simulink model "roundabout_onthego_path"  (R2016b)
settings: Solver=FixedStepAuto  StartTime=0.0  StopTime=inf  RelTol=1e-3
undefined symbols (not defined in the file): DiscIntNeverNeededParam, vehicle_name
libraries: simulink x8, SCANeR_API x6
(part 1 of 2)
settings Model: Creator=z041288  LastModifiedBy=z041288

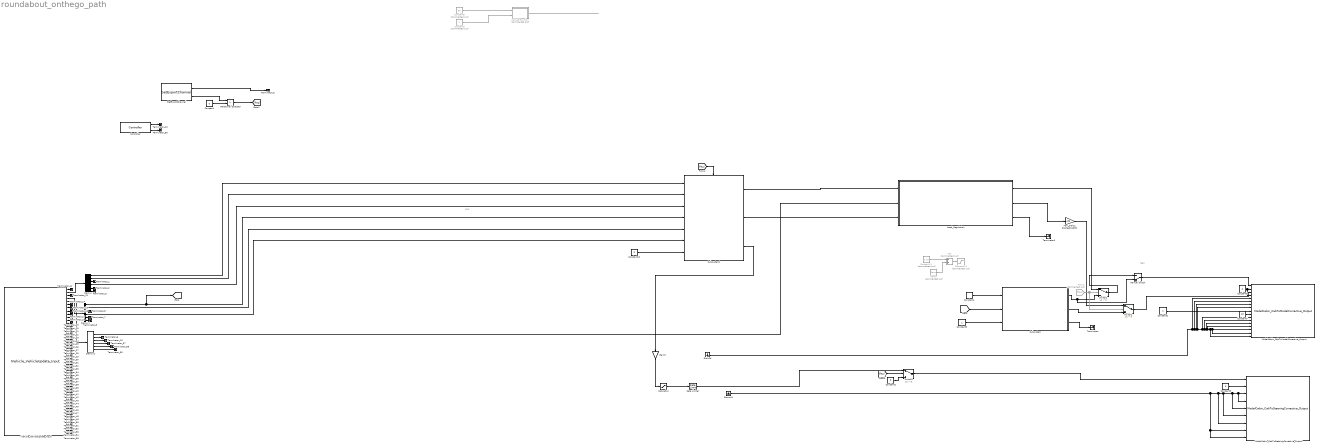
== system roundabout_onthego_path ==
  note: yaw
  note: Man
  Accel_Regulation : Subsystem
  Add : Sum  Commented=on
  Constant{,1,3,6} (4 alike) : Constant  Value=0
  Constant10 : Constant  Value=2
  Constant11 : Constant  Commented=on  Value=2.78
  Constant2 : Constant
  Constant4 : Constant  Value=10*5/18
  Constant5 : Constant
  Constant7 : Constant  Value=10
  Constant8 : Constant  Commented=on  Value=50
  Constant9 : Constant  Commented=on  Value=4
  Controller : SCANeR_API/Controller  Priority=1  Config='NEWCONFIG_Training'  ProcName='SIMULINK'  Frequency=100  NetworkOutputFrequency=100  TimeOut=3000  IsSynchronized=on
  Demux : Demux  Outputs=6
  Demux1 : Demux  Outputs=6
  Demux2 : Demux  Outputs=6
  From2 : From  Commented=on  GotoTag=flag
  Gain3 : Gain  Gain=1/57
  GetExportChannel : SCANeR_API/GetExportChannel  Priority=0  ExportChannelCategory='debug'  ExportChannelName='SF_debug_001'  VehicleId=-1
  Ground : Ground
  Ground1 : Ground
  IVehicle_VehicleUpdate_Input : SCANeR_API/Network inputs/IVehicle/IVehicle_VehicleUpdate_Input  Priority=2  ev=off  vhlId=0
  MATLAB Function : MATLAB Function  Commented=on  TreatAsAtomicUnit=on
  Manual Switch : ManualSwitch  CurrentSetting=0
  Max_brake_SCANeR=400N : Gain  Gain=400
  ModelCabin_CabToModelCorrective_Output : SCANeR_API/SHM outputs/ModelCabin/ModelCabin_CabToModelCorrective_Output  Priority=2  shmId=0
  ModelCabin_CabToSteeringCorrective_Output : SCANeR_API/SHM outputs/ModelCabin/ModelCabin_CabToSteeringCorrective_Output  Priority=2  shmId=0
  Ramp : simulink/Sources/Ramp  Commented=on  slope=25/30  start=0  X0=0
  Rate Limiter : RateLimiter  RisingSlewLimit=10  FallingSlewLimit=-10  SampleTimeMode=inherited
  Relational Operator : RelationalOperator  Operator=>  OutDataTypeStr=boolean  RndMeth=Simplest
  Saturation : Saturate  UpperLimit=10  LowerLimit=-10
  Saturation1 : Saturate  Commented=on  UpperLimit=75/18  LowerLimit=0
  Subsystem : Subsystem
  Subsystem1 : Subsystem
  Switch1 : Switch  Criteria=u2 > Threshold  Threshold=5
  Switch2 : Switch  Criteria=u2 > Threshold
  Switch3 : Switch  Criteria=u2 > Threshold
  Terminator : Terminator
  Terminator1 : Terminator
  Terminator_{1..3,5..59} (58 alike) : Terminator
  wires:
  GetExportChannel/1 -> Terminator_9/1
  GetExportChannel/2 -> Relational Operator/1
  Constant/1 -> Relational Operator/2
  Controller/1 -> Terminator_10/1
  Controller/2 -> Terminator_56/1
  IVehicle_VehicleUpdate_Input/2 -> Demux/1
  IVehicle_VehicleUpdate_Input/4 -> Demux1/1
  Gain3/1 -> Saturation/1
  Ground1/1 -> ModelCabin_CabToSteeringCorrective_Output/8, ModelCabin_CabToSteeringCorrective_Output/9, ModelCabin_CabToSteeringCorrective_Output/4, ModelCabin_CabToSteeringCorrective_Output/3, ModelCabin_CabToSteeringCorrective_Output/5, ModelCabin_CabToSteeringCorrective_Output/6, ModelCabin_CabToSteeringCorrective_Output/7
  Demux/3 -> Terminator_1/1
  Demux/5 -> Terminator_2/1
  Demux/6 -> Terminator_3/1
  Demux1/3 -> Terminator_5/1
  Demux1/5 -> Terminator_7/1
  Demux1/6 -> Terminator_8/1
  IVehicle_VehicleUpdate_Input/1 -> Terminator_11/1
  IVehicle_VehicleUpdate_Input/3 -> Terminator_12/1
  IVehicle_VehicleUpdate_Input/5 -> Demux2/1
  IVehicle_VehicleUpdate_Input/6 -> Terminator_14/1
  IVehicle_VehicleUpdate_Input/7 -> Terminator_15/1
  IVehicle_VehicleUpdate_Input/8 -> Terminator_16/1
  IVehicle_VehicleUpdate_Input/9 -> Terminator_17/1
  IVehicle_VehicleUpdate_Input/10 -> Terminator_18/1
  IVehicle_VehicleUpdate_Input/11 -> Terminator_19/1
  IVehicle_VehicleUpdate_Input/12 -> Terminator_20/1
  IVehicle_VehicleUpdate_Input/13 -> Terminator_21/1
  IVehicle_VehicleUpdate_Input/14 -> Terminator_22/1
  IVehicle_VehicleUpdate_Input/15 -> Terminator_23/1
  IVehicle_VehicleUpdate_Input/16 -> Terminator_24/1
  IVehicle_VehicleUpdate_Input/17 -> Terminator_25/1
  IVehicle_VehicleUpdate_Input/18 -> Terminator_26/1
  IVehicle_VehicleUpdate_Input/19 -> Terminator_27/1
  IVehicle_VehicleUpdate_Input/20 -> Terminator_28/1
  IVehicle_VehicleUpdate_Input/21 -> Terminator_29/1
  IVehicle_VehicleUpdate_Input/22 -> Terminator_30/1
  IVehicle_VehicleUpdate_Input/23 -> Terminator_31/1
  IVehicle_VehicleUpdate_Input/24 -> Terminator_32/1
  IVehicle_VehicleUpdate_Input/25 -> Terminator_33/1
  IVehicle_VehicleUpdate_Input/26 -> Terminator_34/1
  IVehicle_VehicleUpdate_Input/27 -> Terminator_35/1
  IVehicle_VehicleUpdate_Input/28 -> Terminator_36/1
  IVehicle_VehicleUpdate_Input/29 -> Terminator_37/1
  IVehicle_VehicleUpdate_Input/30 -> Terminator_38/1
  IVehicle_VehicleUpdate_Input/31 -> Terminator_39/1
  IVehicle_VehicleUpdate_Input/32 -> Terminator_40/1
  IVehicle_VehicleUpdate_Input/33 -> Terminator_41/1
  IVehicle_VehicleUpdate_Input/34 -> Terminator_42/1
  IVehicle_VehicleUpdate_Input/35 -> Terminator_43/1
  IVehicle_VehicleUpdate_Input/36 -> Terminator_44/1
  IVehicle_VehicleUpdate_Input/37 -> Terminator_45/1
  IVehicle_VehicleUpdate_Input/38 -> Terminator_46/1
  IVehicle_VehicleUpdate_Input/39 -> Terminator_47/1
  IVehicle_VehicleUpdate_Input/40 -> Terminator_48/1
  IVehicle_VehicleUpdate_Input/41 -> Terminator_49/1
  IVehicle_VehicleUpdate_Input/42 -> Terminator_50/1
  IVehicle_VehicleUpdate_Input/43 -> Terminator_51/1
  IVehicle_VehicleUpdate_Input/44 -> Terminator_52/1
  IVehicle_VehicleUpdate_Input/45 -> Terminator_53/1
  IVehicle_VehicleUpdate_Input/46 -> Terminator_54/1
  IVehicle_VehicleUpdate_Input/47 -> Terminator_55/1
  Ground/1 -> ModelCabin_CabToModelCorrective_Output/5, ModelCabin_CabToModelCorrective_Output/6, ModelCabin_CabToModelCorrective_Output/7, ModelCabin_CabToModelCorrective_Output/8, ModelCabin_CabToModelCorrective_Output/11, ModelCabin_CabToModelCorrective_Output/12, ModelCabin_CabToModelCorrective_Output/13, ModelCabin_CabToModelCorrective_Output/14, ModelCabin_CabToModelCorrective_Output/17, ModelCabin_CabToModelCorrective_Output/16, ModelCabin_CabToModelCorrective_Output/15
  Demux1/1 -> Subsystem1/4(xd_in), [speed]  "vlongi"
  Saturation/1 -> Rate Limiter/1
  Demux2/1 -> Accel_Regulation/2(Vehicle_accel_[m/s2])
  Accel_Regulation/2(brake [0_1]) -> Max_brake_SCANeR=400N/1
  Demux2/2 -> Terminator_6/1
  Demux2/3 -> Terminator_13/1
  Demux2/4 -> Terminator_57/1
  Demux2/5 -> Terminator_58/1
  Demux2/6 -> Terminator_59/1
  Constant2/1 -> ModelCabin_CabToModelCorrective_Output/9
  Constant3/1 -> ModelCabin_CabToSteeringCorrective_Output/2
  Constant5/1 -> Subsystem/3(Speed_control_on)
  [speed] -> Subsystem/2(Vehicle_Speed_[m/s])
  Accel_Regulation/1(accel [0_1]) -> Switch1/1
  Subsystem/1(accel_regul [0_1]) -> Manual Switch/2, Switch1/3
  Switch1/1 -> Manual Switch/1
  Constant6/1 -> ModelCabin_CabToModelCorrective_Output/4, ModelCabin_CabToModelCorrective_Output/2
  Constant7/1 -> ModelCabin_CabToModelCorrective_Output/10
  Max_brake_SCANeR=400N/1 -> Switch2/1
  Subsystem/2(Driver_Brake [0_1]) -> Switch2/3
  Switch2/1 -> ModelCabin_CabToModelCorrective_Output/3
  Relational Operator/1 -> [flag]
  From2/1 -> Switch1/2, Switch2/2
  Subsystem/3(Gear_d) -> Terminator/1
  Accel_Regulation/3(Gear_d) -> Terminator1/1
  Demux/1 -> Subsystem1/1(x_in)  "x"
  Demux/2 -> Subsystem1/2(y_in)  "y"
  Demux/4 -> Subsystem1/3(yaw_in)  "yaw"
  Demux1/2 -> Subsystem1/5(yd_in)  "vlat"
  Demux1/4 -> Subsystem1/6(yawd_in)  "yawdot"
  Subsystem1/1(Out11) -> Accel_Regulation/1(Intended_Vehicle_accel_[m/s2])
  Subsystem1/2(Out12) -> Accel_Regulation/3(Accel_control_on)
  Subsystem1/3(Out13) -> Gain3/1
  [flag] -> Subsystem1/Enable
  Rate Limiter/1 -> Switch3/1
  Switch3/1 -> ModelCabin_CabToSteeringCorrective_Output/1
  [flag] -> Switch3/2
  Constant1/1 -> Switch3/3
  Constant9/1 -> MATLAB Function/2(exit)
  Constant8/1 -> MATLAB Function/1(r)
  MATLAB Function/1(y) -> ?
  Constant10/1 -> Subsystem1/7(Maneuver)
  Manual Switch/1 -> ModelCabin_CabToModelCorrective_Output/1
  Ramp/1 -> Add/2
  Add/1 -> Saturation1/1
  Constant11/1 -> Add/1
  Constant4/1 -> Subsystem/1(Intended_Vehicle_Speed_[m/s])

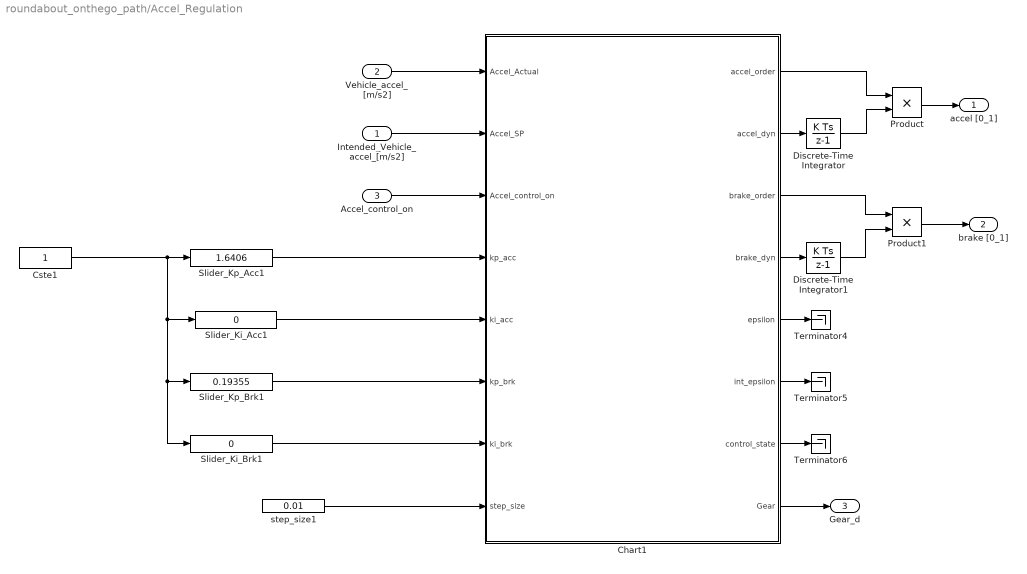
== system roundabout_onthego_path/Accel_Regulation ==
  Intended_Vehicle_accel_[m/s2] : Inport
  Vehicle_accel_[m/s2] : Inport  Port=2
  Accel_control_on : Inport  Port=3
  Chart1 : Stateflow chart  TreatAsAtomicUnit=on  SystemSampleTime=0.01
  Cste1 : Constant  SampleTime=0.01
  Discrete-Time Integrator : DiscreteIntegrator  SampleTime=-1  LimitOutput=on  UpperSaturationLimit=1  LowerSaturationLimit=0  ICPrevOutput=DiscIntNeverNeededParam  ICPrevScaledInput=DiscIntNeverNeededParam
  Discrete-Time Integrator1 : DiscreteIntegrator  SampleTime=-1  LimitOutput=on  UpperSaturationLimit=1  LowerSaturationLimit=0  ICPrevOutput=DiscIntNeverNeededParam  ICPrevScaledInput=DiscIntNeverNeededParam
  Product : Product
  Product1 : Product
  Slider_Ki_Acc1 : simulink/Math Operations/Slider Gain  low=0  gain=0  high=2
  Slider_Ki_Brk1 : simulink/Math Operations/Slider Gain  low=0  gain=0  high=2
  Slider_Kp_Acc1 : simulink/Math Operations/Slider Gain  low=0  gain=1.6406  high=10
  Slider_Kp_Brk1 : simulink/Math Operations/Slider Gain  low=0  gain=0.19355  high=2
  Terminator4 : Terminator
  Terminator5 : Terminator
  Terminator6 : Terminator
  step_size1 : Constant  Value=0.01  SampleTime=0.01
  accel [0_1] : Outport
  brake [0_1] : Outport  Port=2
  Gear_d : Outport  Port=3
  wires:
  Intended_Vehicle_accel_[m/s2]/1 -> Chart1/2(Accel_SP)
  Vehicle_accel_[m/s2]/1 -> Chart1/1(Accel_Actual)
  Accel_control_on/1 -> Chart1/3(Accel_control_on)
  step_size1/1 -> Chart1/8(step_size)
  Chart1/5(epsilon) -> Terminator4/1
  Chart1/6(int_epsilon) -> Terminator5/1
  Slider_Kp_Acc1/1 -> Chart1/4(kp_acc)
  Slider_Ki_Acc1/1 -> Chart1/5(ki_acc)
  Slider_Ki_Brk1/1 -> Chart1/7(ki_brk)
  Slider_Kp_Brk1/1 -> Chart1/6(kp_brk)
  Cste1/1 -> Slider_Ki_Acc1/1, Slider_Kp_Brk1/1, Slider_Ki_Brk1/1, Slider_Kp_Acc1/1
  Chart1/4(brake_dyn) -> Discrete-Time Integrator1/1
  Chart1/2(accel_dyn) -> Discrete-Time Integrator/1
  Chart1/1(accel_order) -> Product/1
  Discrete-Time Integrator/1 -> Product/2
  Product/1 -> accel [0_1]/1
  Chart1/3(brake_order) -> Product1/1
  Discrete-Time Integrator1/1 -> Product1/2
  Product1/1 -> brake [0_1]/1
  Chart1/7(control_state) -> Terminator6/1
  Chart1/8(Gear) -> Gear_d/1

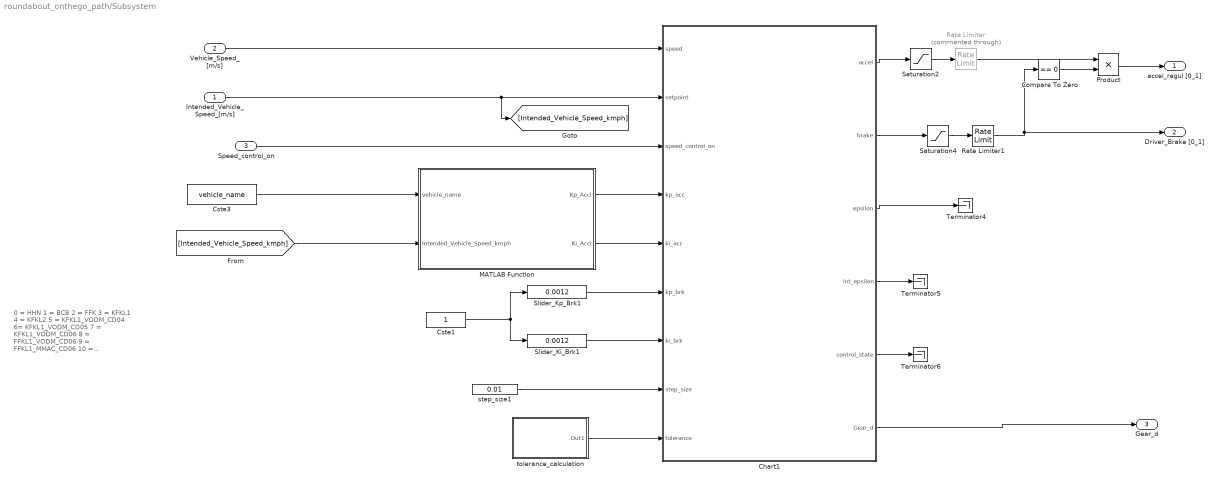
== system roundabout_onthego_path/Subsystem ==
  note: 0 = HHN
      | 1 = BCB
      | 2 = FFK
      | 3 = KFKL1
      | 4 = KFKL2
      | 5 = KFKL1_VODM_CD04
      | 6= KFKL1_VODM_CD05
      | 7 = KFKL1_VODM_CD06
      | 8 = FFKL1_VODM_CD06
      | 9 = FFKL1_MMAC_CD06
      | 10 = FFKL2_MMAC_CD06
      | 11 = KFKL2_MMAC_CD06
      | 12 = XDD_35T_TRS_L2H2
  Intended_Vehicle_Speed_[m/s] : Inport
  Vehicle_Speed_[m/s] : Inport  Port=2
  Speed_control_on : Inport  Port=3
  Chart1 : Stateflow chart  TreatAsAtomicUnit=on  SystemSampleTime=0.01
  Compare To Zero : simulink/Logic and Bit Operations/Compare To Zero  relop===  OutDataTypeStr=boolean
  Cste1 : Constant  SampleTime=0.01
  Cste3 : Constant  Value=vehicle_name  SampleTime=0.01
  MATLAB Function : MATLAB Function  TreatAsAtomicUnit=on
  Product : Product
  Rate Limiter : RateLimiter  Commented=through  RisingSlewLimit=0.5  SampleTimeMode=inherited
  Rate Limiter1 : RateLimiter  RisingSlewLimit=0.2  SampleTimeMode=inherited
  Saturation2 : Saturate  UpperLimit=1  LowerLimit=0  SampleTime=0.01
  Saturation4 : Saturate  UpperLimit=1  LowerLimit=0  SampleTime=0.01
  Slider_Ki_Brk1 : simulink/Math Operations/Slider Gain  low=0  gain=0.0012  high=2
  Slider_Kp_Brk1 : simulink/Math Operations/Slider Gain  low=0  gain=0.0012  high=1
  Terminator4 : Terminator
  Terminator5 : Terminator
  Terminator6 : Terminator
  step_size1 : Constant  Value=0.01  SampleTime=0.01
  tolerance_calculation : Subsystem
  accel_regul [0_1] : Outport
  Driver_Brake [0_1] : Outport  Port=2
  Gear_d : Outport  Port=3
  wires:
  Cste1/1 -> Slider_Kp_Brk1/1, Slider_Ki_Brk1/1
  Slider_Kp_Brk1/1 -> Chart1/6(kp_brk)
  Slider_Ki_Brk1/1 -> Chart1/7(ki_brk)
  MATLAB Function/2(Ki_Accl) -> Chart1/5(ki_acc)
  MATLAB Function/1(Kp_Accl) -> Chart1/4(kp_acc)
  Chart1/5(control_state) -> Terminator6/1
  Chart1/4(int_epsilon) -> Terminator5/1
  Chart1/3(epsilon) -> Terminator4/1
  Chart1/2(brake) -> Saturation4/1
  step_size1/1 -> Chart1/8(step_size)
  Saturation4/1 -> Rate Limiter1/1
  Vehicle_Speed_[m/s]/1 -> Chart1/1(speed)
  Intended_Vehicle_Speed_[m/s]/1 -> [Intended_Vehicle_Speed_kmph], Chart1/2(setpoint)
  Saturation2/1 -> Rate Limiter/1
  Rate Limiter/1 -> Product/1
  Product/1 -> accel_regul [0_1]/1
  Rate Limiter1/1 -> Compare To Zero/1, Driver_Brake [0_1]/1
  Chart1/6(Gear_d) -> Gear_d/1
  Speed_control_on/1 -> Chart1/3(speed_control_on)
  Cste3/1 -> MATLAB Function/1(vehicle_name)
  [Intended_Vehicle_Speed_kmph] -> MATLAB Function/2(Intended_Vehicle_Speed_kmph)
  Compare To Zero/1 -> Product/2
  Chart1/1(accel) -> Saturation2/1
  tolerance_calculation/1(Out1) -> Chart1/9(tolerance)

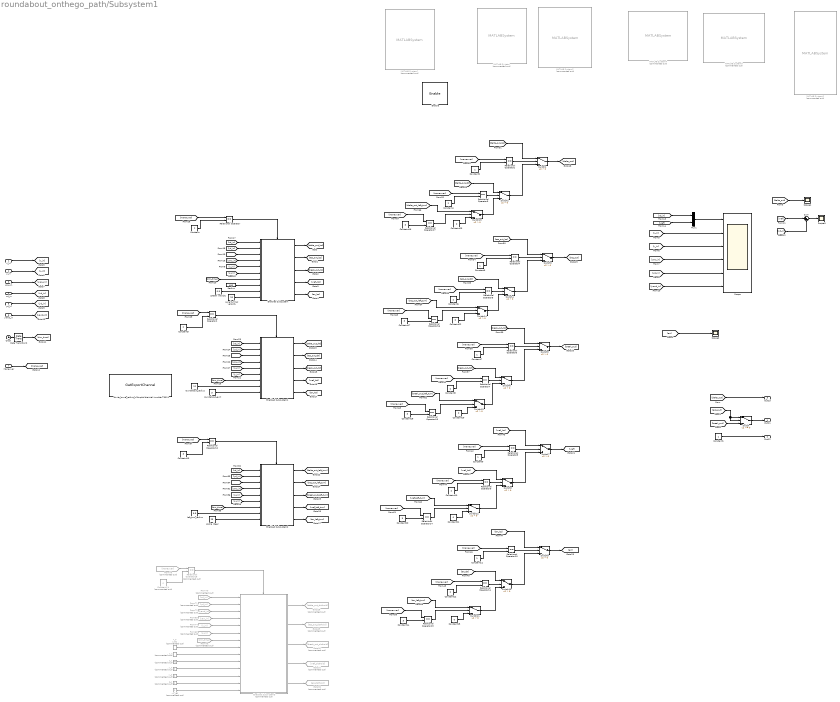
== system roundabout_onthego_path/Subsystem1 ==
  x_in : Inport
  y_in : Inport  Port=2
  yaw_in : Inport  Port=3
  xd_in : Inport  Port=4
  yd_in : Inport  Port=5
  yawd_in : Inport  Port=6
  Maneuver : Inport  Port=7
  Enable : EnablePort  PropagateVarSize=During execution
  Clock : Clock
  Constant{,1..2,5,7,9,11} (7 alike) : Constant
  Constant{3..4,6,8,10,12} (6 alike) : Constant  Value=2
  Constant{13..14,16..18,20} (6 alike) : Constant  Value=3
  Constant{15,19,21..23} (5 alike) : Constant  Value=0
  Constant24 : Constant  Commented=on  Value=4
  Enabled Subsystem : Subsystem  TreatAsAtomicUnit=on
  Enabled Subsystem1 : Subsystem  TreatAsAtomicUnit=on
  Enabled Subsystem2 : Subsystem  TreatAsAtomicUnit=on
  Enabled Subsystem3 : Subsystem  Commented=on  TreatAsAtomicUnit=on
  From68 : From  Commented=on  GotoTag=y_in
  From69 : From  Commented=on  GotoTag=yaw_in
  From70 : From  Commented=on  GotoTag=xd_in
  From71 : From  Commented=on  GotoTag=yd_in
  From72 : From  Commented=on  GotoTag=yawd_in
  From73 : From  Commented=on  GotoTag=sim_time
  From74 : From  Commented=on  GotoTag=x_in
  From75 : From  Commented=on  GotoTag=maneuver
  Goto28 : Goto  Commented=on  GotoTag=delta_out_clothoid
  Goto29 : Goto  Commented=on  GotoTag=acc_out_clothoid
  Goto30 : Goto  Commented=on  GotoTag=break_out_clothoid
  Goto31 : Goto  Commented=on  GotoTag=vref_clothoid
  Goto32 : Goto  Commented=on  GotoTag=err_clothoid
  Lateral velocity : Constant  Value=0.5
  Longitudinal velocity : Constant  Value=20
  MATLAB System : MATLABSystem  Commented=on  System=casadi_block_MPCtry_1  SimulateUsing=Interpreted execution
      mask Type: casadi_block_MPCtry_1
      mask Display:
      | disp('casadi_block_MPCtry_1');
      | port_label('input',1,'xd_in');
      | port_label('input',2,'yd_in');
      | port_label('input',3,'yawd_in');
      | port_label('input',4,'yaw_in');
      | port_label('input',5,'x_in');
      | port_label('input',6,'y_in');
      | port_label('input',7,'t');
      | port_label('output',1,'delta_out');
      | port_label('output',2,'acc_out');
      | port_label('output',3,'break_out');
      | port_label('output',4,'vref');
      | port_label('output',5,'err');
  MATLAB System1 : MATLABSystem  Commented=on  System=casadi_block_MPCtry_3  SimulateUsing=Interpreted execution
      mask Type: casadi_block_MPCtry_3
      mask Display:
      | disp('casadi_block_MPCtry_3');
      | port_label('input',1,'xd_in');
      | port_label('input',2,'yd_in');
      | port_label('input',3,'yawd_in');
      | port_label('input',4,'yaw_in');
      | port_label('input',5,'x_in');
      | port_label('input',6,'y_in');
      | port_label('input',7,'t');
      | port_label('output',1,'delta_out');
      | port_label('output',2,'acc_out');
      | port_label('output',3,'break_out');
      | port_label('output',4,'vref');
      | port_label('output',5,'err');
  MATLAB System2 : MATLABSystem  Commented=on  System=casadi_block_MPC_LSS  SimulateUsing=Interpreted execution
      mask Type: casadi_block_MPC_LSS
      mask Display:
      | disp('casadi_block_MPC_LSS');
      | port_label('input',1,'xd_in');
      | port_label('input',2,'yd_in');
      | port_label('input',3,'yawd_in');
      | port_label('input',4,'yaw_in');
      | port_label('input',5,'x_in');
      | port_label('input',6,'y_in');
      | port_label('input',7,'t');
      | port_label('output',1,'delta_out');
      | port_label('output',2,'acc_out');
      | port_label('output',3,'break_out');
      | port_label('output',4,'vref');
      | port_label('output',5,'err');
  MATLAB System3 : MATLABSystem  Commented=on  System=casadi_block_MPC_left_turn  SimulateUsing=Interpreted execution
      mask Type: casadi_block_MPC_left_turn
      mask Display:
      | disp('casadi_block_MPC_left_turn');
      | port_label('input',1,'xd_in');
      | port_label('input',2,'yd_in');
      | port_label('input',3,'yawd_in');
      | port_label('input',4,'yaw_in');
      | port_label('input',5,'x_in');
      | port_label('input',6,'y_in');
      | port_label('input',7,'t');
      | port_label('output',1,'delta_out');
      | port_label('output',2,'acc_out');
      | port_label('output',3,'break_out');
      | port_label('output',4,'vref');
      | port_label('output',5,'err');
  MATLAB System4 : MATLABSystem  Commented=on  System=casadi_block_MPC_left_turn_2  SimulateUsing=Interpreted execution
      mask Type: casadi_block_MPC_left_turn_2
      mask Display:
      | disp('casadi_block_MPC_left_turn_2');
      | port_label('input',1,'xd_in');
      | port_label('input',2,'yd_in');
      | port_label('input',3,'yawd_in');
      | port_label('input',4,'yaw_in');
      | port_label('input',5,'x_in');
      | port_label('input',6,'y_in');
      | port_label('input',7,'t');
      | port_label('output',1,'delta_out');
      | port_label('output',2,'acc_out');
      | port_label('output',3,'break_out');
      | port_label('output',4,'vref');
      | port_label('output',5,'err');
  MATLAB System5 : MATLABSystem  Commented=on  System=casadi_block_MPCtry_4  SimulateUsing=Interpreted execution
      mask Type: casadi_block_MPCtry_4
      mask Display:
      | disp('casadi_block_MPCtry_4');
      | port_label('input',1,'xd_in');
      | port_label('input',2,'yd_in');
      | port_label('input',3,'yawd_in');
      | port_label('input',4,'yaw_in');
      | port_label('input',5,'x_in');
      | port_label('input',6,'y_in');
      | port_label('input',7,'t');
      | port_label('input',8,'ref_path');
      | port_label('output',1,'delta_out');
      | port_label('output',2,'acc_out');
      | port_label('output',3,'break_out');
      | port_label('output',4,'vref');
      | port_label('output',5,'err');
  Mux1 : Mux  Inputs=2
  Radius : Constant  Value=400
  Rate Transition2 : RateTransition  OutPortSampleTime=0.02
  Relational Operator{,1..17} (18 alike) : RelationalOperator  Operator===  OutDataTypeStr=boolean  RndMeth=Simplest
  Relational Operator18 : RelationalOperator  Commented=on  Operator===  OutDataTypeStr=boolean  RndMeth=Simplest
  Scope : Scope  NumInputPorts=6
  Scope1 : Scope
  Scope2 : Scope
  Scope3 : Scope
  Sum : Sum  Inputs=|+-
  Switch : Switch
  Switch{1..15} (15 alike) : Switch  Criteria=u2 > Threshold
  alpha (deg) : Constant  Value=23
  driver_curve_radius_m export channel number - 6011 : SCANeR_API/GetExportChannel  Priority=0  ExportChannelCategory='system'  ExportChannelName='driver_curve_radius_m'  VehicleId=-1
  left_turn_radius : Constant  Value=9.5
  roundabout_exit : Constant  Value=3
  roundabout_radius : Constant  Value=12
  t_o : Constant  Commented=on
  t_s : Constant  Commented=on  Value=90
  vv_ref : Constant  Commented=on
  x_o : Constant  Commented=on
  x_s : Constant  Commented=on  Value=1.82
  y_o : Constant  Commented=on
  y_s : Constant  Commented=on  Value=-60
  Out11 : Outport
  Out12 : Outport  Port=2
  Out13 : Outport  Port=3
  wires:
  [x_in] -> Scope/2
  [y_in] -> Scope/3
  [yawd_in] -> Scope/6
  [yd_in] -> Scope/5
  [err] -> Scope2/1
  Rate Transition2/1 -> [sim_time]
  Mux1/1 -> Scope/1
  [acc_out] -> Switch/2, Switch/1
  Clock/1 -> Rate Transition2/1
  [yaw_in] -> Scope/4
  Switch/1 -> Out11/1
  [break_out] -> Switch/3
  Sum/1 -> Scope3/1
  Constant1/1 -> Out12/1
  roundabout_radius/1 -> Enabled Subsystem1/8(In8)
  roundabout_exit/1 -> Enabled Subsystem1/9(In9)
  Enabled Subsystem/1(Out1) -> [delta_out_lss]
  Enabled Subsystem/2(Out2) -> [acc_out_lss]
  Enabled Subsystem/3(Out3) -> [break_out_lss]
  Enabled Subsystem/4(Out4) -> [vref_lss]
  Enabled Subsystem/5(Out5) -> [err_lss]
  x_in/1 -> [x_in]
  y_in/1 -> [y_in]
  yaw_in/1 -> [yaw_in]
  xd_in/1 -> [xd_in]
  yd_in/1 -> [yd_in]
  yawd_in/1 -> [yawd_in]
  [vref] -> Sum/1
  [xd_in] -> Sum/2
  [xd_in] -> Mux1/1
  [vref] -> Mux1/2
  [delta_out] -> Out13/1
  [x_in] -> Enabled Subsystem/5(In5)
  [y_in] -> Enabled Subsystem/6(In6)
  [yaw_in] -> Enabled Subsystem/4(In4)
  [xd_in] -> Enabled Subsystem/1(In1)
  [yd_in] -> Enabled Subsystem/2(In2)
  [yawd_in] -> Enabled Subsystem/3(In3)
  [sim_time] -> Enabled Subsystem/7(In7)
  [x_in] -> Enabled Subsystem1/5(In5)
  [y_in] -> Enabled Subsystem1/6(In6)
  [yaw_in] -> Enabled Subsystem1/4(In4)
  [xd_in] -> Enabled Subsystem1/1(In1)
  [yd_in] -> Enabled Subsystem1/2(In2)
  [yawd_in] -> Enabled Subsystem1/3(In3)
  [sim_time] -> Enabled Subsystem1/7(In7)
  Maneuver/1 -> [maneuver]
  [maneuver] -> Relational Operator/1
  Constant/1 -> Relational Operator/2
  Constant3/1 -> Relational Operator1/2
  [maneuver] -> Relational Operator1/1
  Relational Operator/1 -> Enabled Subsystem/Enable
  Relational Operator1/1 -> Enabled Subsystem1/Enable
  Enabled Subsystem1/1(Out1) -> [delta_out_rbt]
  Enabled Subsystem1/2(Out2) -> [acc_out_rbt]
  Enabled Subsystem1/3(Out3) -> [break_out_rbt]
  Enabled Subsystem1/4(Out4) -> [vref_rbt]
  Enabled Subsystem1/5(Out5) -> [err_rbt]
  [maneuver] -> Relational Operator2/1
  Constant2/1 -> Relational Operator2/2
  Relational Operator2/1 -> Switch1/2
  [delta_out_lss] -> Switch1/1
  [maneuver] -> Relational Operator3/1
  Constant4/1 -> Relational Operator3/2
  Relational Operator3/1 -> Switch2/2
  Switch2/1 -> Switch1/3
  [delta_out_rbt] -> Switch2/1
  Switch1/1 -> [delta_out]
  [maneuver] -> Relational Operator4/1
  Constant5/1 -> Relational Operator4/2
  Relational Operator4/1 -> Switch3/2
  [acc_out_lss] -> Switch3/1
  [maneuver] -> Relational Operator5/1
  Constant6/1 -> Relational Operator5/2
  Relational Operator5/1 -> Switch4/2
  Switch4/1 -> Switch3/3
  [acc_out_rbt] -> Switch4/1
  Switch3/1 -> [acc_out]
  [maneuver] -> Relational Operator6/1
  Constant7/1 -> Relational Operator6/2
  Relational Operator6/1 -> Switch5/2
  [break_out_lss] -> Switch5/1
  [maneuver] -> Relational Operator7/1
  Constant8/1 -> Relational Operator7/2
  Relational Operator7/1 -> Switch6/2
  Switch6/1 -> Switch5/3
  [break_out_rbt] -> Switch6/1
  Switch5/1 -> [break_out]
  [maneuver] -> Relational Operator8/1
  Constant9/1 -> Relational Operator8/2
  Relational Operator8/1 -> Switch7/2
  [vref_lss] -> Switch7/1
  [maneuver] -> Relational Operator9/1
  Constant10/1 -> Relational Operator9/2
  Relational Operator9/1 -> Switch8/2
  Switch8/1 -> Switch7/3
  [vref_rbt] -> Switch8/1
  Switch7/1 -> [vref]
  [maneuver] -> Relational Operator10/1
  Constant11/1 -> Relational Operator10/2
  Relational Operator10/1 -> Switch9/2
  [err_lss] -> Switch9/1
  [maneuver] -> Relational Operator11/1
  Constant12/1 -> Relational Operator11/2
  Relational Operator11/1 -> Switch10/2
  Switch10/1 -> Switch9/3
  [err_rbt] -> Switch10/1
  Switch9/1 -> [err]
  Radius/1 -> Enabled Subsystem/8(In8)
  Lateral velocity/1 -> Enabled Subsystem/9(In9)
  Longitudinal velocity/1 -> Enabled Subsystem/10(In10)
  Switch15/1 -> Switch2/3
  Switch14/1 -> Switch4/3
  Switch13/1 -> Switch6/3
  Switch12/1 -> Switch8/3
  Switch11/1 -> Switch10/3
  [delta_out] -> Scope1/1
  left_turn_radius/1 -> Enabled Subsystem2/8(In8)
  alpha (deg)/1 -> Enabled Subsystem2/9(In9)
  [x_in] -> Enabled Subsystem2/5(In5)
  [y_in] -> Enabled Subsystem2/6(In6)
  [yaw_in] -> Enabled Subsystem2/4(In4)
  [xd_in] -> Enabled Subsystem2/1(In1)
  [yd_in] -> Enabled Subsystem2/2(In2)
  [yawd_in] -> Enabled Subsystem2/3(In3)
  [sim_time] -> Enabled Subsystem2/7(In7)
  Constant13/1 -> Relational Operator12/2
  [maneuver] -> Relational Operator12/1
  Relational Operator12/1 -> Enabled Subsystem2/Enable
  Enabled Subsystem2/1(Out1) -> [delta_out_left_turn]
  Enabled Subsystem2/2(Out2) -> [acc_out_left_turn]
  Enabled Subsystem2/3(Out3) -> [break_out_left_turn]
  Enabled Subsystem2/4(Out4) -> [vref_left_turn]
  Enabled Subsystem2/5(Out5) -> [err_left_turn]
  [maneuver] -> Relational Operator13/1
  Constant14/1 -> Relational Operator13/2
  Relational Operator13/1 -> Switch11/2
  [err_left_turn] -> Switch11/1
  Constant15/1 -> Switch11/3
  [maneuver] -> Relational Operator14/1
  Relational Operator14/1 -> Switch12/2
  [vref_left_turn] -> Switch12/1
  Constant21/1 -> Switch12/3
  Constant20/1 -> Relational Operator14/2
  [maneuver] -> Relational Operator15/1
  Relational Operator15/1 -> Switch13/2
  [break_out_left_turn] -> Switch13/1
  Constant19/1 -> Switch13/3
  Constant18/1 -> Relational Operator15/2
  [maneuver] -> Relational Operator16/1
  Relational Operator16/1 -> Switch14/2
  [acc_out_left_turn] -> Switch14/1
  Constant22/1 -> Switch14/3
  Constant17/1 -> Relational Operator16/2
  [maneuver] -> Relational Operator17/1
  Relational Operator17/1 -> Switch15/2
  [delta_out_left_turn] -> Switch15/1
  Constant23/1 -> Switch15/3
  Constant16/1 -> Relational Operator17/2
  x_s/1 -> Enabled Subsystem3/8(In8)
  y_s/1 -> Enabled Subsystem3/9(In9)
  From74/1 -> Enabled Subsystem3/5(In5)
  From68/1 -> Enabled Subsystem3/6(In6)
  From69/1 -> Enabled Subsystem3/4(In4)
  From70/1 -> Enabled Subsystem3/1(In1)
  From71/1 -> Enabled Subsystem3/2(In2)
  From72/1 -> Enabled Subsystem3/3(In3)
  From73/1 -> Enabled Subsystem3/7(In7)
  Constant24/1 -> Relational Operator18/2
  From75/1 -> Relational Operator18/1
  Relational Operator18/1 -> Enabled Subsystem3/Enable
  Enabled Subsystem3/1(Out1) -> Goto28/1
  Enabled Subsystem3/2(Out2) -> Goto29/1
  Enabled Subsystem3/3(Out3) -> Goto30/1
  Enabled Subsystem3/4(Out4) -> Goto31/1
  Enabled Subsystem3/5(Out5) -> Goto32/1
  t_s/1 -> Enabled Subsystem3/10(In10)
  x_o/1 -> Enabled Subsystem3/11(In11)
  y_o/1 -> Enabled Subsystem3/12(In12)
  t_o/1 -> Enabled Subsystem3/13(In13)
  vv_ref/1 -> Enabled Subsystem3/14(In14)

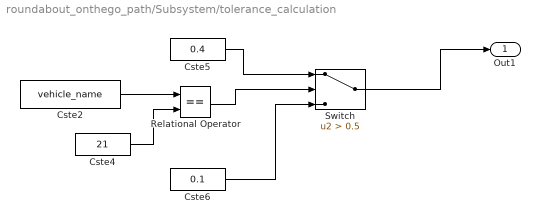
== system roundabout_onthego_path/Subsystem/tolerance_calculation ==
  Cste2 : Constant  Value=vehicle_name  SampleTime=0.01
  Cste4 : Constant  Value=21  SampleTime=0.01
  Cste5 : Constant  Value=0.4  SampleTime=0.01
  Cste6 : Constant  Value=0.1  SampleTime=0.01
  Relational Operator : RelationalOperator  Operator===  OutDataTypeStr=boolean  RndMeth=Simplest
  Switch : Switch  Criteria=u2 > Threshold  Threshold=0.5
  Out1 : Outport
  wires:
  Switch/1 -> Out1/1
  Cste6/1 -> Switch/3
  Cste5/1 -> Switch/1
  Cste2/1 -> Relational Operator/1
  Cste4/1 -> Relational Operator/2
  Relational Operator/1 -> Switch/2

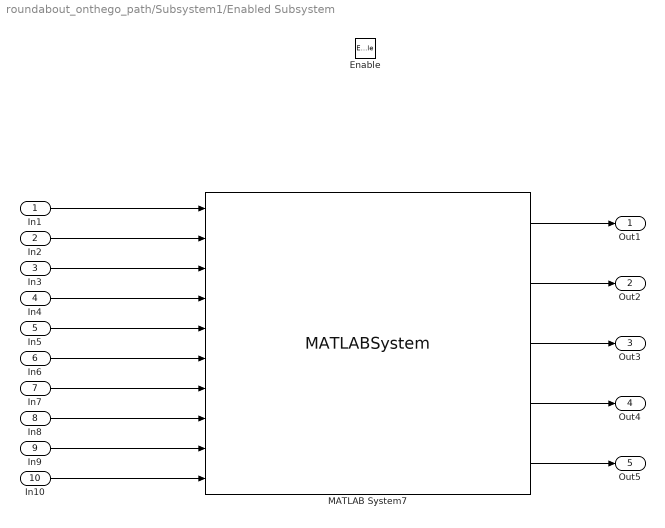
== system roundabout_onthego_path/Subsystem1/Enabled Subsystem ==
  In1 : Inport
  In2 : Inport  Port=2
  In3 : Inport  Port=3
  In4 : Inport  Port=4
  In5 : Inport  Port=5
  In6 : Inport  Port=6
  In7 : Inport  Port=7
  In8 : Inport  Port=8
  In9 : Inport  Port=9
  In10 : Inport  Port=10
  Enable : EnablePort
  MATLAB System7 : MATLABSystem  System=casadi_block_MPC_LSS_onthego  SimulateUsing=Interpreted execution
      mask Type: casadi_block_MPC_LSS_onthego
      mask Display:
      | disp('casadi_block_MPC_LSS_onthego');
      | port_label('input',1,'xd_in');
      | port_label('input',2,'yd_in');
      | port_label('input',3,'yawd_in');
      | port_label('input',4,'yaw_in');
      | port_label('input',5,'x_in');
      | port_label('input',6,'y_in');
      | port_label('input',7,'t');
      | port_label('input',8,'R');
      | port_label('input',9,'vlat_ref');
      | port_label('input',10,'vlongi_ref');
      | port_label('output',1,'delta_out');
      | port_label('output',2,'acc_out');
      | port_label('output',3,'break_out');
      | port_label('output',4,'vref');
      | port_label('output',5,'err');
  Out1 : Outport
  Out2 : Outport  Port=2
  Out3 : Outport  Port=3
  Out4 : Outport  Port=4
  Out5 : Outport  Port=5
  wires:
  In1/1 -> MATLAB System7/1
  In2/1 -> MATLAB System7/2
  In3/1 -> MATLAB System7/3
  In4/1 -> MATLAB System7/4
  In5/1 -> MATLAB System7/5
  In7/1 -> MATLAB System7/7
  In6/1 -> MATLAB System7/6
  MATLAB System7/1 -> Out1/1
  MATLAB System7/2 -> Out2/1
  MATLAB System7/3 -> Out3/1
  MATLAB System7/4 -> Out4/1
  MATLAB System7/5 -> Out5/1
  In10/1 -> MATLAB System7/10
  In9/1 -> MATLAB System7/9
  In8/1 -> MATLAB System7/8

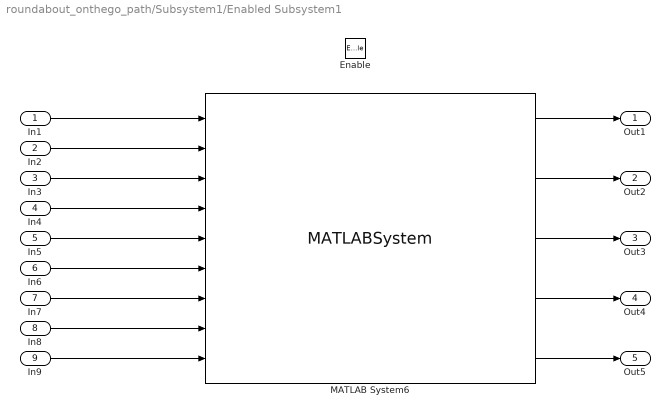
== system roundabout_onthego_path/Subsystem1/Enabled Subsystem1 ==
  In1 : Inport
  In2 : Inport  Port=2
  In3 : Inport  Port=3
  In4 : Inport  Port=4
  In5 : Inport  Port=5
  In6 : Inport  Port=6
  In7 : Inport  Port=7
  In8 : Inport  Port=8
  In9 : Inport  Port=9
  Enable : EnablePort
  MATLAB System6 : MATLABSystem  System=casadi_block_MPCtry_5  SimulateUsing=Interpreted execution
      mask Type: casadi_block_MPCtry_5
      mask Display:
      | disp('casadi_block_MPCtry_5');
      | port_label('input',1,'xd_in');
      | port_label('input',2,'yd_in');
      | port_label('input',3,'yawd_in');
      | port_label('input',4,'yaw_in');
      | port_label('input',5,'x_in');
      | port_label('input',6,'y_in');
      | port_label('input',7,'t');
      | port_label('input',8,'r');
      | port_label('input',9,'ex');
      | port_label('output',1,'delta_out');
      | port_label('output',2,'acc_out');
      | port_label('output',3,'break_out');
      | port_label('output',4,'vref');
      | port_label('output',5,'err');
  Out1 : Outport
  Out2 : Outport  Port=2
  Out3 : Outport  Port=3
  Out4 : Outport  Port=4
  Out5 : Outport  Port=5
  wires:
  In1/1 -> MATLAB System6/1
  In2/1 -> MATLAB System6/2
  In3/1 -> MATLAB System6/3
  In4/1 -> MATLAB System6/4
  In5/1 -> MATLAB System6/5
  In7/1 -> MATLAB System6/7
  In6/1 -> MATLAB System6/6
  In9/1 -> MATLAB System6/9
  In8/1 -> MATLAB System6/8
  MATLAB System6/1 -> Out1/1
  MATLAB System6/2 -> Out2/1
  MATLAB System6/3 -> Out3/1
  MATLAB System6/4 -> Out4/1
  MATLAB System6/5 -> Out5/1

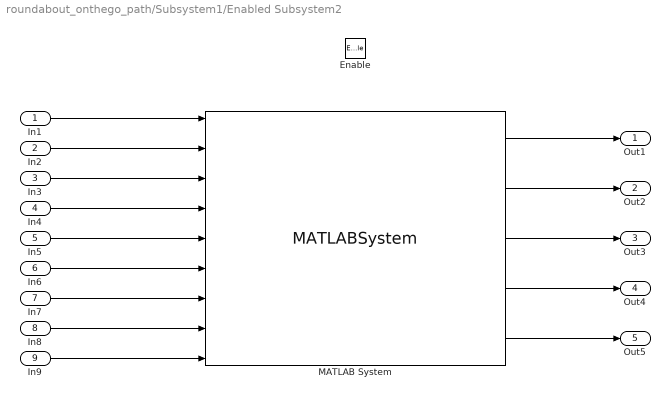
== system roundabout_onthego_path/Subsystem1/Enabled Subsystem2 ==
  In1 : Inport
  In2 : Inport  Port=2
  In3 : Inport  Port=3
  In4 : Inport  Port=4
  In5 : Inport  Port=5
  In6 : Inport  Port=6
  In7 : Inport  Port=7
  In8 : Inport  Port=8
  In9 : Inport  Port=9
  Enable : EnablePort
  MATLAB System : MATLABSystem  System=casadi_block_MPC_left_turn_onthego  SimulateUsing=Interpreted execution
      mask Type: casadi_block_MPC_left_turn_onthego
      mask Display:
      | disp('casadi_block_MPC_left_turn_onthego');
      | port_label('input',1,'xd_in');
      | port_label('input',2,'yd_in');
      | port_label('input',3,'yawd_in');
      | port_label('input',4,'yaw_in');
      | port_label('input',5,'x_in');
      | port_label('input',6,'y_in');
      | port_label('input',7,'t');
      | port_label('input',8,'r');
      | port_label('input',9,'alpha');
      | port_label('output',1,'delta_out');
      | port_label('output',2,'acc_out');
      | port_label('output',3,'break_out');
      | port_label('output',4,'vref');
      | port_label('output',5,'err');
  Out1 : Outport
  Out2 : Outport  Port=2
  Out3 : Outport  Port=3
  Out4 : Outport  Port=4
  Out5 : Outport  Port=5
  wires:
  In1/1 -> MATLAB System/1
  In2/1 -> MATLAB System/2
  In3/1 -> MATLAB System/3
  In4/1 -> MATLAB System/4
  In5/1 -> MATLAB System/5
  In7/1 -> MATLAB System/7
  In6/1 -> MATLAB System/6
  In9/1 -> MATLAB System/9
  In8/1 -> MATLAB System/8
  MATLAB System/1 -> Out1/1
  MATLAB System/2 -> Out2/1
  MATLAB System/3 -> Out3/1
  MATLAB System/4 -> Out4/1
  MATLAB System/5 -> Out5/1

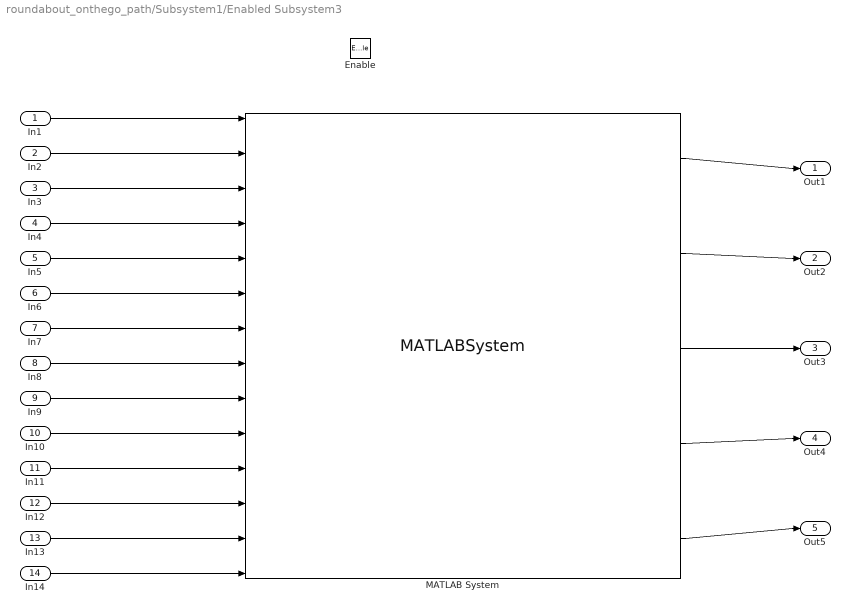
== system roundabout_onthego_path/Subsystem1/Enabled Subsystem3 ==
  In1 : Inport
  In2 : Inport  Port=2
  In3 : Inport  Port=3
  In4 : Inport  Port=4
  In5 : Inport  Port=5
  In6 : Inport  Port=6
  In7 : Inport  Port=7
  In8 : Inport  Port=8
  In9 : Inport  Port=9
  In10 : Inport  Port=10
  In11 : Inport  Port=11
  In12 : Inport  Port=12
  In13 : Inport  Port=13
  In14 : Inport  Port=14
  Enable : EnablePort
  MATLAB System : MATLABSystem  System=casadi_block_MPC_track_clothoid_onthego  SimulateUsing=Interpreted execution
      mask Type: casadi_block_MPC_track_clothoid_onthego
      mask Display:
      | disp('casadi_block_MPC_track_clothoid_onthego');
      | port_label('input',1,'xd_in');
      | port_label('input',2,'yd_in');
      | port_label('input',3,'yawd_in');
      | port_label('input',4,'yaw_in');
      | port_label('input',5,'x_in');
      | port_label('input',6,'y_in');
      | port_label('input',7,'t');
      | port_label('input',8,'x_s_in');
      | port_label('input',9,'y_s_in');
      | port_label('input',10,'t_s_in');
      | port_label('input',11,'x_s_out');
      | port_label('input',12,'y_s_out');
      | port_label('input',13,'t_s_out');
      | port_label('input',14,'vv_ref');
      | port_label('output',1,'delta_out');
      | port_label('output',2,'acc_out');
      | port_label('output',3,'break_out');
      | port_label('output',4,'vref');
      | port_label('output',5,'err');
  Out1 : Outport
  Out2 : Outport  Port=2
  Out3 : Outport  Port=3
  Out4 : Outport  Port=4
  Out5 : Outport  Port=5
  wires:
  In1/1 -> MATLAB System/1
  In2/1 -> MATLAB System/2
  In3/1 -> MATLAB System/3
  In4/1 -> MATLAB System/4
  In5/1 -> MATLAB System/5
  In7/1 -> MATLAB System/7
  In6/1 -> MATLAB System/6
  In9/1 -> MATLAB System/9
  In8/1 -> MATLAB System/8
  MATLAB System/1 -> Out1/1
  MATLAB System/2 -> Out2/1
  MATLAB System/3 -> Out3/1
  MATLAB System/4 -> Out4/1
  MATLAB System/5 -> Out5/1
  In10/1 -> MATLAB System/10
  In11/1 -> MATLAB System/11
  In12/1 -> MATLAB System/12
  In13/1 -> MATLAB System/13
  In14/1 -> MATLAB System/14

== stateflow chart roundabout_onthego_path/Accel_Regulation/Chart1 ==
  state Accel_Control/
    state Control_Off/
      accel_order= 0;
      brake_order= 0;
      accel_dyn= 0;
      brake_dyn= 0;
      int_epsilon = 0;
      Gear=10;
    state Controller/
      limit_accel = 1/kp_acc;
      limit_brake = 1/kp_brk;
      state Acceleration_regulation/
        state accel/
          control_state = 2;
          accel_order=1;
          brake_order= 0;
          accel_dyn=  kp_acc*epsilon + ki_acc*int_epsilon;
          brake_dyn= 0;
          Gear=10;
        (junction 59) -> accel [order 1] : [abs(epsilon) < limit_accel & control_state == 2]
            | {int_epsilon = int_epsilon + step_size*epsilon;}
        (junction 59) -> accel [order 2] : {int_epsilon = 0;}
      state Brake_regulation/
        state brake/
          control_state = 1;
          accel_order=0;
          brake_order=1;
          accel_dyn= 0;
          brake_dyn=  kp_brk*epsilon + ki_brk*int_epsilon;
          Gear=10;
        (junction 101) -> brake [order 1] : [abs(epsilon) < limit_brake & control_state == 1]
            | {int_epsilon = int_epsilon + step_size*epsilon;}
        (junction 101) -> brake [order 2] : {int_epsilon = 0;}
      accel -> (junction 56)
      brake -> (junction 56)
      (junction 56) -> (junction 59) [order 1] : [Accel_SP >= 0]
          | {epsilon =Accel_SP-Accel_Actual;}
      (junction 56) -> (junction 101) [order 2] : {epsilon =Accel_Actual-Accel_SP;}
    (default) -> (junction 55)
    (junction 55) -> Control_Off [order 1] : [Accel_control_on == 0]
    Control_Off -> (junction 55)
    Controller -> (junction 55) : [Accel_control_on == 0]
    (junction 55) -> (junction 56) [order 2] : {control_state = 0;}
  data: Accel_Actual input double; Accel_SP input double; Accel_control_on input double; accel_order output double; accel_dyn output double; brake_order output double; brake_dyn output double; kp_acc input double; ki_acc input double; kp_brk input double; ki_brk input double; step_size input double; limit_accel local double; limit_brake local double; epsilon output double; int_epsilon output double; control_state output double; Gear output double
